simulink library "csc_sei_sensonor_external_imu_lib"  (R2014b)
settings: Solver=ode45  StartTime=0.0  StopTime=10.0  RelTol=1e-3
libraries: util_common_lib x2, util_info_lib x1, csu_imk_imu_kinematis_lib x1, csu_snm_sensonor_noise_model_lib x1
settings Model: Creator=escrane  LastModifiedBy=mstewart

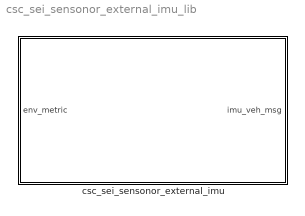
== system csc_sei_sensonor_external_imu_lib ==
  csc_sei_sensonor_external_imu : Subsystem

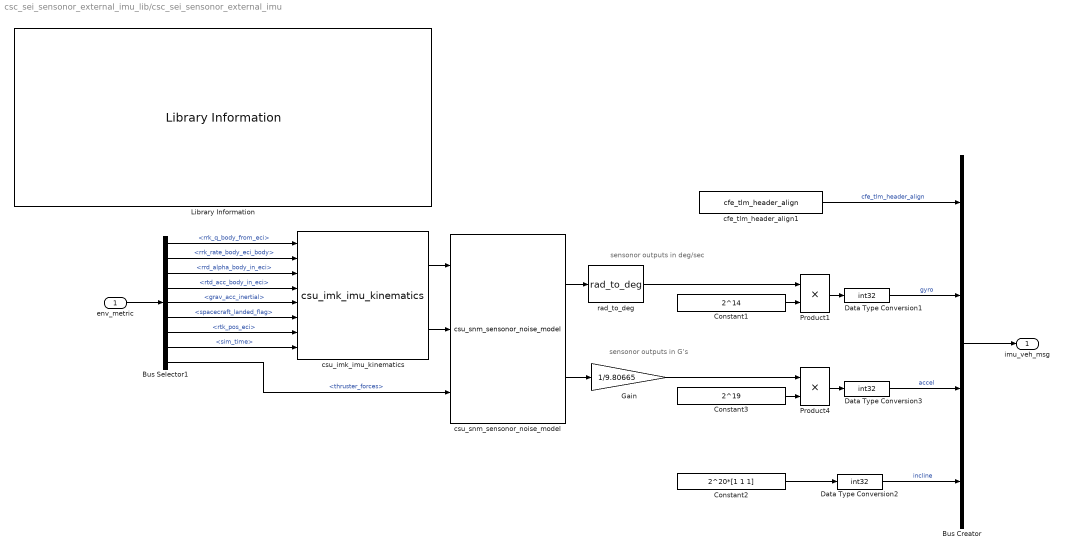
== system csc_sei_sensonor_external_imu_lib/csc_sei_sensonor_external_imu ==
  note: sensonor outputs in deg/sec
  note: sensonor outputs in G's
  env_metric : Inport
  Bus Creator : BusCreator  OutDataTypeStr=Bus: imu_veh_msg  NonVirtualBus=on
  Bus Selector1 : BusSelector  OutputSignals=lander_state_bus.rrk_q_body_from_eci,lander_state_bus.rrk_rate_body_eci_body,lander_state_bus.rrd_alpha_body_in_eci,lander_state_bus.rtd_acc_body_in_eci,enf_force_torque_msg.grav_acc_inertial,lander_state_bus.spacecraft_landed_flag,lander_state_bus.rtk_pos_eci,sim_time,actuator_mtv_msg.thruster_forces
  Constant1 : Constant  Value=2^14  OutDataTypeStr=double
  Constant2 : Constant  Value=2^20*[1 1 1]  OutDataTypeStr=double
  Constant3 : Constant  Value=2^19  OutDataTypeStr=double
  Data Type Conversion1 : DataTypeConversion  OutDataTypeStr=int32  RndMeth=Round
  Data Type Conversion2 : DataTypeConversion  OutDataTypeStr=int32  RndMeth=Round
  Data Type Conversion3 : DataTypeConversion  OutDataTypeStr=int32  RndMeth=Round
  Gain : Gain  Gain=1/9.80665
  Library Information : util_info_lib/Library Information  owner='escrane'
  Product1 : Product  Inputs=**  OutDataTypeStr=double  RndMeth=Zero
  Product4 : Product  Inputs=**  OutDataTypeStr=double  RndMeth=Zero
  cfe_tlm_header_align1 : util_common_lib/cfe_tlm_header_align
  csu_imk_imu_kinematics : csu_imk_imu_kinematis_lib/csu_imk_imu_kinematics  imu_position=sei_position  imu_dcm=sei_dcm
  csu_snm_sensonor_noise_model : csu_snm_sensonor_noise_model_lib/csu_snm_sensonor_noise_model
  rad_to_deg : util_common_lib/rad_to_deg  SystemSampleTime=-1
  imu_veh_msg : Outport
  wires:
  Gain/1 -> Product4/1
  rad_to_deg/1 -> Product1/1
  csu_snm_sensonor_noise_model/1 -> rad_to_deg/1
  csu_snm_sensonor_noise_model/2 -> Gain/1
  cfe_tlm_header_align1/1 -> Bus Creator/1  "cfe_tlm_header_align"
  Bus Creator/1 -> imu_veh_msg/1
  Data Type Conversion1/1 -> Bus Creator/2  "gyro"
  Product1/1 -> Data Type Conversion1/1
  Constant1/1 -> Product1/2
  Product4/1 -> Data Type Conversion3/1
  Constant3/1 -> Product4/2
  csu_imk_imu_kinematics/1 -> csu_snm_sensonor_noise_model/1
  csu_imk_imu_kinematics/2 -> csu_snm_sensonor_noise_model/2
  Bus Selector1/2 -> csu_imk_imu_kinematics/2  "<rrk_rate_body_eci_body>"
  Bus Selector1/3 -> csu_imk_imu_kinematics/3  "<rrd_alpha_body_in_eci>"
  Bus Selector1/4 -> csu_imk_imu_kinematics/4  "<rtd_acc_body_in_eci>"
  Bus Selector1/5 -> csu_imk_imu_kinematics/5  "<grav_acc_inertial>"
  Data Type Conversion3/1 -> Bus Creator/3  "accel"
  Bus Selector1/1 -> csu_imk_imu_kinematics/1  "<rrk_q_body_from_eci>"
  env_metric/1 -> Bus Selector1/1
  Bus Selector1/6 -> csu_imk_imu_kinematics/6  "<spacecraft_landed_flag>"
  Bus Selector1/7 -> csu_imk_imu_kinematics/7  "<rtk_pos_eci>"
  Bus Selector1/8 -> csu_imk_imu_kinematics/8  "<sim_time>"
  Bus Selector1/9 -> csu_snm_sensonor_noise_model/3  "<thruster_forces>"
  Constant2/1 -> Data Type Conversion2/1
  Data Type Conversion2/1 -> Bus Creator/4  "incline"
